simulink model "BuildingHeatLoadCalc"  (R2026a)
settings: Solver=ode1be  StopTime=31532400  FixedStep=3600  AbsTol=1e-3
undefined symbols (not defined in the file): BuildingThermalLib, lib_BuildingThermal
libraries: ExternalWall_lib x47, WallSelector_lib x36, fl_lib x32, RoomWithAirVolume x15, nesl_utility x4, TemperatureSource_lib x1, DayScheduler_lib x1, SolarRadiationAtLocation_lib x1
(part 5 of 5)

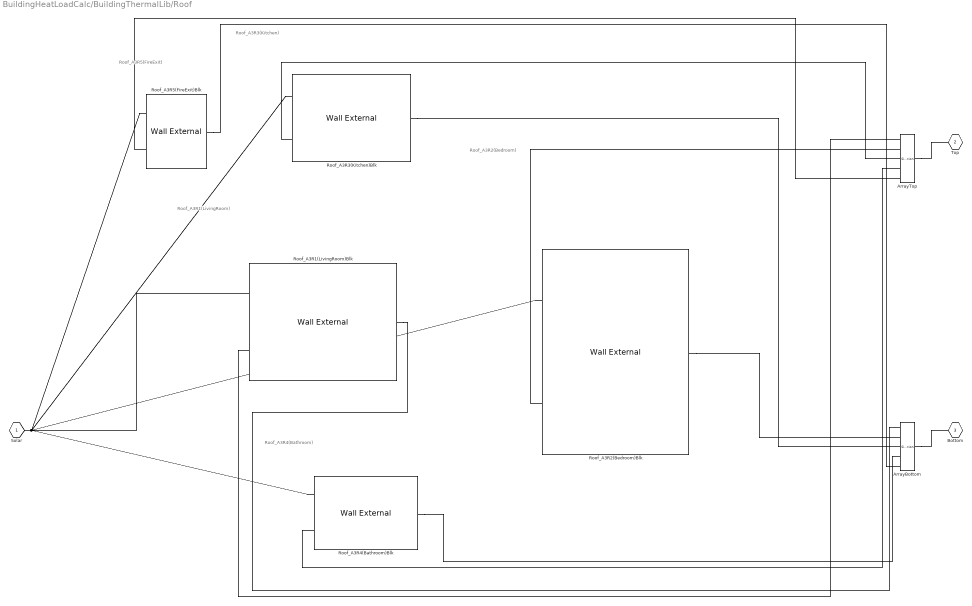
== system BuildingHeatLoadCalc/BuildingThermalLib/Roof ==
  note: Roof_A3R1(LivingRoom)
  note: Roof_A3R2(Bedroom)
  note: Roof_A3R3(Kitchen)
  note: Roof_A3R4(Bathroom)
  note: Roof_A3R5(FireExit)
  ArrayBottom : SimscapeArrayConnection  Domain=foundation.thermal.thermal  ConcatenateDimension=1  NumScalarElements=5
  ArrayTop : SimscapeArrayConnection  Domain=foundation.thermal.thermal  ConcatenateDimension=1  NumScalarElements=5
  Roof_A3R1(LivingRoom)Blk : ExternalWall_lib/Wall External  extWallModel=wallExternalModelOption.wallSolar  wallLength=2.4384 % Parameterized on : 09-Jun-2026 19:35:13 m  wallHeight=3.048 % Parameterized on : 09-Jun-2026 19:35:13 m  wallThickness=0.04 % Parameterized on : 09-Jun-2026 19:35:13 m  wallMaterialDen=2000 % Parameterized on : 09-Jun-2026 19:35:15 kg/m^3  wallMaterialCp=1100 % Parameterized on : 09-Jun-2026 19:35:15 J/(K*kg)  wallAbsorptivity=0.6 % Parameterized on : 09-Jun-2026 19:35:15  wallThermalK=1.4 % Parameterized on : 09-Jun-2026 19:35:15 W/(K*m)  winLength=1 m  winHeight=0.5 m  winThickness=0.007 m  winMaterialDen=2500 kg/m^3  winMaterialCp=787 J/(K*kg)  winAbsorptivity=0.35  winThermalK=1 W/(K*m)  winTransmissivity=0.45  ventLength=0.1 m  ventHeight=0.1 m  extToWallHTC=20 % Parameterized on : 09-Jun-2026 19:35:15 W/(K*m^2)  intToRoomHTC=30 % Parameterized on : 09-Jun-2026 19:35:15 W/(K*m^2)  iniT=275.8 % Parameterized on : 09-Jun-2026 19:38:28 K  latitude=47.376 % Parameterized on : 09-Jun-2026 19:38:30  longitude=8.541 % Parameterized on : 09-Jun-2026 19:38:30  localTime=15.00 % Parameterized on : 09-Jun-2026 19:38:30  dayLightS=0 % Parameterized on : 09-Jun-2026 19:38:30  surfAngle=0 % Parameterized on : 09-Jun-2026 19:35:13 deg  surfUnitV=[0,-1] % Parameterized on : 09-Jun-2026 19:35:13  startYear=2024 % Parameterized on : 09-Jun-2026 19:38:30  startMonth=1 % Parameterized on : 09-Jun-2026 19:38:30  startDay=1 % Parameterized on : 09-Jun-2026 19:38:30  startHr=1 % Parameterized on : 09-Jun-2026 19:38:30  numHrsData=8760 % Parameterized on : 09-Jun-2026 19:38:30  interp_method=simscape.enum.interpolation.linear  extrap_method=simscape.enum.extrapolation.nearest
  Roof_A3R2(Bedroom)Blk : ExternalWall_lib/Wall External  extWallModel=wallExternalModelOption.wallSolar  wallLength=4.2672 % Parameterized on : 09-Jun-2026 19:35:13 m  wallHeight=3.048 % Parameterized on : 09-Jun-2026 19:35:13 m  wallThickness=0.04 % Parameterized on : 09-Jun-2026 19:35:13 m  wallMaterialDen=2000 % Parameterized on : 09-Jun-2026 19:35:15 kg/m^3  wallMaterialCp=1100 % Parameterized on : 09-Jun-2026 19:35:15 J/(K*kg)  wallAbsorptivity=0.6 % Parameterized on : 09-Jun-2026 19:35:15  wallThermalK=1.4 % Parameterized on : 09-Jun-2026 19:35:15 W/(K*m)  winLength=1 m  winHeight=0.5 m  winThickness=0.007 m  winMaterialDen=2500 kg/m^3  winMaterialCp=787 J/(K*kg)  winAbsorptivity=0.35  winThermalK=1 W/(K*m)  winTransmissivity=0.45  ventLength=0.1 m  ventHeight=0.1 m  extToWallHTC=20 % Parameterized on : 09-Jun-2026 19:35:15 W/(K*m^2)  intToRoomHTC=30 % Parameterized on : 09-Jun-2026 19:35:15 W/(K*m^2)  iniT=275.8 % Parameterized on : 09-Jun-2026 19:38:28 K  latitude=47.376 % Parameterized on : 09-Jun-2026 19:38:30  longitude=8.541 % Parameterized on : 09-Jun-2026 19:38:30  localTime=15.00 % Parameterized on : 09-Jun-2026 19:38:30  dayLightS=0 % Parameterized on : 09-Jun-2026 19:38:30  surfAngle=0 % Parameterized on : 09-Jun-2026 19:35:13 deg  surfUnitV=[0,-1] % Parameterized on : 09-Jun-2026 19:35:13  startYear=2024 % Parameterized on : 09-Jun-2026 19:38:30  startMonth=1 % Parameterized on : 09-Jun-2026 19:38:30  startDay=1 % Parameterized on : 09-Jun-2026 19:38:30  startHr=1 % Parameterized on : 09-Jun-2026 19:38:30  numHrsData=8760 % Parameterized on : 09-Jun-2026 19:38:30  interp_method=simscape.enum.interpolation.linear  extrap_method=simscape.enum.extrapolation.nearest
  Roof_A3R3(Kitchen)Blk : ExternalWall_lib/Wall External  extWallModel=wallExternalModelOption.wallSolar  wallLength=1.8288 % Parameterized on : 09-Jun-2026 19:35:13 m  wallHeight=2.4384 % Parameterized on : 09-Jun-2026 19:35:13 m  wallThickness=0.04 % Parameterized on : 09-Jun-2026 19:35:13 m  wallMaterialDen=2000 % Parameterized on : 09-Jun-2026 19:35:15 kg/m^3  wallMaterialCp=1100 % Parameterized on : 09-Jun-2026 19:35:15 J/(K*kg)  wallAbsorptivity=0.6 % Parameterized on : 09-Jun-2026 19:35:15  wallThermalK=1.4 % Parameterized on : 09-Jun-2026 19:35:15 W/(K*m)  winLength=1 m  winHeight=0.5 m  winThickness=0.007 m  winMaterialDen=2500 kg/m^3  winMaterialCp=787 J/(K*kg)  winAbsorptivity=0.35  winThermalK=1 W/(K*m)  winTransmissivity=0.45  ventLength=0.1 m  ventHeight=0.1 m  extToWallHTC=20 % Parameterized on : 09-Jun-2026 19:35:15 W/(K*m^2)  intToRoomHTC=30 % Parameterized on : 09-Jun-2026 19:35:15 W/(K*m^2)  iniT=275.8 % Parameterized on : 09-Jun-2026 19:38:28 K  latitude=47.376 % Parameterized on : 09-Jun-2026 19:38:30  longitude=8.541 % Parameterized on : 09-Jun-2026 19:38:30  localTime=15.00 % Parameterized on : 09-Jun-2026 19:38:30  dayLightS=0 % Parameterized on : 09-Jun-2026 19:38:30  surfAngle=0 % Parameterized on : 09-Jun-2026 19:35:13 deg  surfUnitV=[0,-1] % Parameterized on : 09-Jun-2026 19:35:13  startYear=2024 % Parameterized on : 09-Jun-2026 19:38:30  startMonth=1 % Parameterized on : 09-Jun-2026 19:38:30  startDay=1 % Parameterized on : 09-Jun-2026 19:38:30  startHr=1 % Parameterized on : 09-Jun-2026 19:38:30  numHrsData=8760 % Parameterized on : 09-Jun-2026 19:38:30  interp_method=simscape.enum.interpolation.linear  extrap_method=simscape.enum.extrapolation.nearest
  Roof_A3R4(Bathroom)Blk : ExternalWall_lib/Wall External  extWallModel=wallExternalModelOption.wallSolar  wallLength=1.524 % Parameterized on : 09-Jun-2026 19:35:13 m  wallHeight=2.1336 % Parameterized on : 09-Jun-2026 19:35:13 m  wallThickness=0.04 % Parameterized on : 09-Jun-2026 19:35:13 m  wallMaterialDen=2000 % Parameterized on : 09-Jun-2026 19:35:15 kg/m^3  wallMaterialCp=1100 % Parameterized on : 09-Jun-2026 19:35:15 J/(K*kg)  wallAbsorptivity=0.6 % Parameterized on : 09-Jun-2026 19:35:15  wallThermalK=1.4 % Parameterized on : 09-Jun-2026 19:35:15 W/(K*m)  winLength=1 m  winHeight=0.5 m  winThickness=0.007 m  winMaterialDen=2500 kg/m^3  winMaterialCp=787 J/(K*kg)  winAbsorptivity=0.35  winThermalK=1 W/(K*m)  winTransmissivity=0.45  ventLength=0.1 m  ventHeight=0.1 m  extToWallHTC=20 % Parameterized on : 09-Jun-2026 19:35:15 W/(K*m^2)  intToRoomHTC=30 % Parameterized on : 09-Jun-2026 19:35:15 W/(K*m^2)  iniT=275.8 % Parameterized on : 09-Jun-2026 19:38:28 K  latitude=47.376 % Parameterized on : 09-Jun-2026 19:38:30  longitude=8.541 % Parameterized on : 09-Jun-2026 19:38:30  localTime=15.00 % Parameterized on : 09-Jun-2026 19:38:30  dayLightS=0 % Parameterized on : 09-Jun-2026 19:38:30  surfAngle=0 % Parameterized on : 09-Jun-2026 19:35:13 deg  surfUnitV=[0,-1] % Parameterized on : 09-Jun-2026 19:35:13  startYear=2024 % Parameterized on : 09-Jun-2026 19:38:30  startMonth=1 % Parameterized on : 09-Jun-2026 19:38:30  startDay=1 % Parameterized on : 09-Jun-2026 19:38:30  startHr=1 % Parameterized on : 09-Jun-2026 19:38:30  numHrsData=8760 % Parameterized on : 09-Jun-2026 19:38:30  interp_method=simscape.enum.interpolation.linear  extrap_method=simscape.enum.extrapolation.nearest
  Roof_A3R5(FireExit)Blk : ExternalWall_lib/Wall External  extWallModel=wallExternalModelOption.wallSolar  wallLength=1.524 % Parameterized on : 09-Jun-2026 19:35:13 m  wallHeight=1.2192 % Parameterized on : 09-Jun-2026 19:35:13 m  wallThickness=0.04 % Parameterized on : 09-Jun-2026 19:35:13 m  wallMaterialDen=2000 % Parameterized on : 09-Jun-2026 19:35:15 kg/m^3  wallMaterialCp=1100 % Parameterized on : 09-Jun-2026 19:35:15 J/(K*kg)  wallAbsorptivity=0.6 % Parameterized on : 09-Jun-2026 19:35:15  wallThermalK=1.4 % Parameterized on : 09-Jun-2026 19:35:15 W/(K*m)  winLength=1 m  winHeight=0.5 m  winThickness=0.007 m  winMaterialDen=2500 kg/m^3  winMaterialCp=787 J/(K*kg)  winAbsorptivity=0.35  winThermalK=1 W/(K*m)  winTransmissivity=0.45  ventLength=0.1 m  ventHeight=0.1 m  extToWallHTC=20 % Parameterized on : 09-Jun-2026 19:35:15 W/(K*m^2)  intToRoomHTC=30 % Parameterized on : 09-Jun-2026 19:35:15 W/(K*m^2)  iniT=275.8 % Parameterized on : 09-Jun-2026 19:38:28 K  latitude=47.376 % Parameterized on : 09-Jun-2026 19:38:30  longitude=8.541 % Parameterized on : 09-Jun-2026 19:38:30  localTime=15.00 % Parameterized on : 09-Jun-2026 19:38:30  dayLightS=0 % Parameterized on : 09-Jun-2026 19:38:30  surfAngle=0 % Parameterized on : 09-Jun-2026 19:35:13 deg  surfUnitV=[0,-1] % Parameterized on : 09-Jun-2026 19:35:13  startYear=2024 % Parameterized on : 09-Jun-2026 19:38:30  startMonth=1 % Parameterized on : 09-Jun-2026 19:38:30  startDay=1 % Parameterized on : 09-Jun-2026 19:38:30  startHr=1 % Parameterized on : 09-Jun-2026 19:38:30  numHrsData=8760 % Parameterized on : 09-Jun-2026 19:38:30  interp_method=simscape.enum.interpolation.linear  extrap_method=simscape.enum.extrapolation.nearest
  Solar : PMIOPort  Side=Left
  Top : PMIOPort  Port=2  Side=Left
  Bottom : PMIOPort  Port=3  Side=Right
  connections:
  Roof_A3R1(LivingRoom)Blk/LConn1 -- Roof_A3R2(Bedroom)Blk/LConn1 -- Roof_A3R3(Kitchen)Blk/LConn1 -- Roof_A3R4(Bathroom)Blk/LConn1 -- Solar/RConn1 -- Roof_A3R5(FireExit)Blk/LConn1
  ArrayTop/RConn1 -- Top/RConn1
  Roof_A3R1(LivingRoom)Blk/LConn2 -- ArrayTop/LConn1
  Roof_A3R2(Bedroom)Blk/LConn2 -- ArrayTop/LConn2
  Roof_A3R3(Kitchen)Blk/LConn2 -- ArrayTop/LConn3
  Roof_A3R4(Bathroom)Blk/LConn2 -- ArrayTop/LConn4
  Roof_A3R5(FireExit)Blk/LConn2 -- ArrayTop/LConn5
  ArrayBottom/RConn1 -- Bottom/RConn1
  Roof_A3R1(LivingRoom)Blk/RConn1 -- ArrayBottom/LConn1
  Roof_A3R2(Bedroom)Blk/RConn1 -- ArrayBottom/LConn2
  Roof_A3R3(Kitchen)Blk/RConn1 -- ArrayBottom/LConn3
  Roof_A3R4(Bathroom)Blk/RConn1 -- ArrayBottom/LConn4
  Roof_A3R5(FireExit)Blk/RConn1 -- ArrayBottom/LConn5

== system BuildingHeatLoadCalc/BuildingThermalLib/roomT ==
  concat1 : fl_lib/Physical Signals/Functions/PS Concatenate  catColumns=true
  concat2 : fl_lib/Physical Signals/Functions/PS Concatenate  catColumns=true
  1 : PMIOPort  Side=Left
  2 : PMIOPort  Port=2  Side=Left
  3 : PMIOPort  Port=3  Side=Left
  v : PMIOPort  Port=4  Side=Right
  connections:
  1/RConn1 -- concat1/LConn1
  2/RConn1 -- concat1/LConn2
  concat1/RConn1 -- concat2/LConn1
  3/RConn1 -- concat2/LConn2
  concat2/RConn1 -- v/RConn1

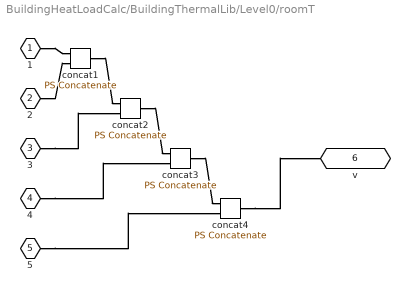
== system BuildingHeatLoadCalc/BuildingThermalLib/Level0/roomT ==
  concat{1..4} (4 alike) : fl_lib/Physical Signals/Functions/PS Concatenate  catColumns=true
  1 : PMIOPort  Side=Left
  2 : PMIOPort  Port=2  Side=Left
  3 : PMIOPort  Port=3  Side=Left
  4 : PMIOPort  Port=4  Side=Left
  5 : PMIOPort  Port=5  Side=Left
  v : PMIOPort  Port=6  Side=Right
  connections:
  1/RConn1 -- concat1/LConn1
  2/RConn1 -- concat1/LConn2
  concat1/RConn1 -- concat2/LConn1
  3/RConn1 -- concat2/LConn2
  concat2/RConn1 -- concat3/LConn1
  4/RConn1 -- concat3/LConn2
  concat3/RConn1 -- concat4/LConn1
  5/RConn1 -- concat4/LConn2
  concat4/RConn1 -- v/RConn1

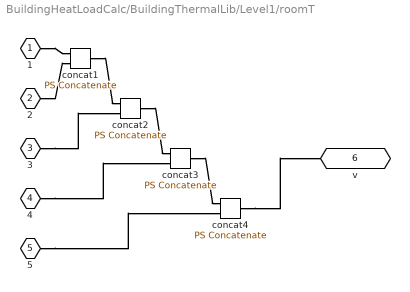
== system BuildingHeatLoadCalc/BuildingThermalLib/Level1/roomT ==
  concat{1..4} (4 alike) : fl_lib/Physical Signals/Functions/PS Concatenate  catColumns=true
  1 : PMIOPort  Side=Left
  2 : PMIOPort  Port=2  Side=Left
  3 : PMIOPort  Port=3  Side=Left
  4 : PMIOPort  Port=4  Side=Left
  5 : PMIOPort  Port=5  Side=Left
  v : PMIOPort  Port=6  Side=Right
  connections:
  1/RConn1 -- concat1/LConn1
  2/RConn1 -- concat1/LConn2
  concat1/RConn1 -- concat2/LConn1
  3/RConn1 -- concat2/LConn2
  concat2/RConn1 -- concat3/LConn1
  4/RConn1 -- concat3/LConn2
  concat3/RConn1 -- concat4/LConn1
  5/RConn1 -- concat4/LConn2
  concat4/RConn1 -- v/RConn1

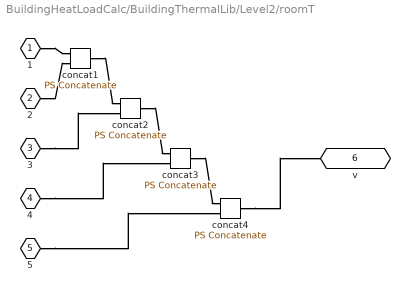
== system BuildingHeatLoadCalc/BuildingThermalLib/Level2/roomT ==
  concat{1..4} (4 alike) : fl_lib/Physical Signals/Functions/PS Concatenate  catColumns=true
  1 : PMIOPort  Side=Left
  2 : PMIOPort  Port=2  Side=Left
  3 : PMIOPort  Port=3  Side=Left
  4 : PMIOPort  Port=4  Side=Left
  5 : PMIOPort  Port=5  Side=Left
  v : PMIOPort  Port=6  Side=Right
  connections:
  1/RConn1 -- concat1/LConn1
  2/RConn1 -- concat1/LConn2
  concat1/RConn1 -- concat2/LConn1
  3/RConn1 -- concat2/LConn2
  concat2/RConn1 -- concat3/LConn1
  4/RConn1 -- concat3/LConn2
  concat3/RConn1 -- concat4/LConn1
  5/RConn1 -- concat4/LConn2
  concat4/RConn1 -- v/RConn1
